simulink model "example_"  (Simulink 6.2)
settings: Solver=ode3  StartTime=0.0  StopTime=10.0  FixedStep=0.05  RelTol=1e-3
libraries: ScienceStimHasomed x1, SyncBlock x1
settings Model: LastModifiedBy=bsaunder
settings DebuggingCC: SolverPrmCheckMsg=warning

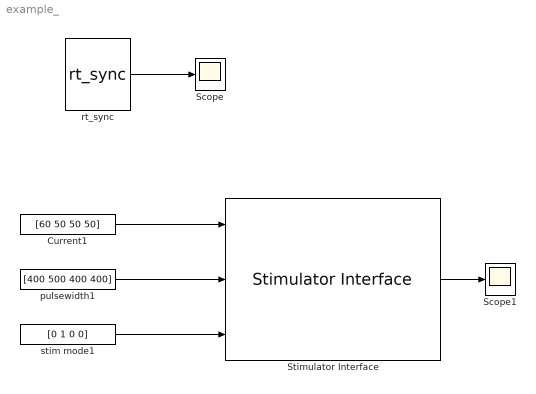
== system example_ ==
  Current1 : Constant  Value=[60 50 50 50]
  Scope : Scope
  Scope1 : Scope
  Stimulator Interface : ScienceStimHasomed/Stimulator Interface  Ts=0.05  com_port=COM2  channelstim=[1 3 5 6]  tsone=15  tstwo=4  channellf=[]  nfactor=[]
  pulsewidth1 : Constant  Value=[400 500 400 400]
  rt_sync : SyncBlock/rt_sync  Ts=0.05
  stim mode1 : Constant  Value=[0 1 0 0]
  wires:
  rt_sync/1 -> Scope/1
  Stimulator Interface/1 -> Scope1/1
  Current1/1 -> Stimulator Interface/1
  pulsewidth1/1 -> Stimulator Interface/2
  stim mode1/1 -> Stimulator Interface/3
